simulink model "cartesian_reg"  (Simulink 8.7)
settings: Solver=ode45  StartTime=0.0  StopTime=T  MaxStep=0.01  RelTol=1e-3
values from neighbouring files (symbols this model uses):
  theta_0 = 0    [init.m]
  x_0 = 2    [init.m]
  y_0 = 0    [init.m]
undefined symbols (not defined in the file or in its folder): cart_reg
settings Model: Creator=marilena  LastModifiedBy=giuseppe  ExtModeAutoUpdateStatusClock=off
settings DataIOCC: SignalLoggingSaveFormat=ModelDataLogs
settings OptimizationCC: ExpressionDepthLimit=2147483647
settings DebuggingCC: SaveWithParameterizedLinksMsg=none  SolverPrmCheckMsg=warning  FcnCallInpInsideContextMsg=UseLocalSettings  StateNameClashWarn=warning  StrictBusMsg=Warning
settings HardwareCC: TargetHWDeviceType=32-bit Generic
settings GRTTargetCC: TargetFcnLib=ansi_tfl_tmw.mat  GeneratePreprocessorConditionals=Use local settings  CombineOutputUpdateFcns=off  GRTInterface=on

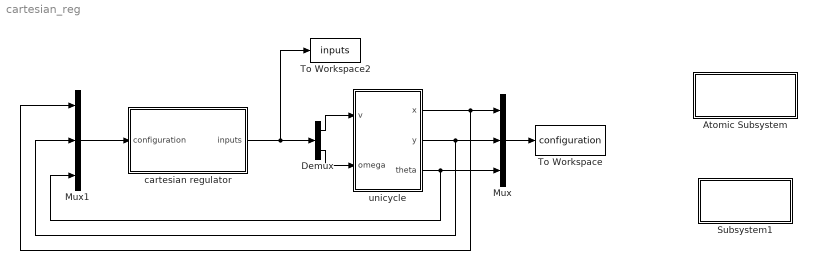
== system cartesian_reg ==
  Atomic Subsystem : Subsystem  TreatAsAtomicUnit=on
      settings: OpenFcn=init
      mask Display: disp('initialization')
  Demux : Demux  Outputs=2
  Mux : Mux  Inputs=3
  Mux1 : Mux  Inputs=3
  Subsystem1 : Subsystem
      settings: OpenFcn=plots
      mask Display: disp('plots')
  To Workspace : ToWorkspace  VariableName=configuration  SaveFormat=Structure With Time  SampleTime=-1
  To Workspace2 : ToWorkspace  VariableName=inputs  SaveFormat=Structure With Time  SampleTime=-1
  cartesian regulator : Subsystem
  unicycle : Subsystem
  wires:
  Mux/1 -> To Workspace/1
  unicycle/3(theta) -> Mux/3, Mux1/3
  unicycle/1(x) -> Mux/1, Mux1/1
  Mux1/1 -> cartesian regulator/1(configuration)
  cartesian regulator/1(inputs) -> Demux/1, To Workspace2/1
  unicycle/2(y) -> Mux/2, Mux1/2
  Demux/1 -> unicycle/1(v)
  Demux/2 -> unicycle/2(omega)

== system cartesian_reg/Atomic Subsystem ==

== system cartesian_reg/Subsystem1 ==

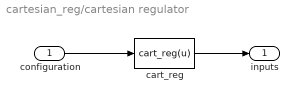
== system cartesian_reg/cartesian regulator ==
  configuration : Inport
  cart_reg : MATLABFcn  Tag={'prova'}  Description=cartesian regulator  MATLABFcn=cart_reg(u)  Output1D=off
  inputs : Outport
  wires:
  configuration/1 -> cart_reg/1
  cart_reg/1 -> inputs/1

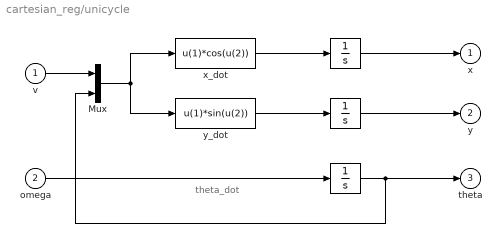
== system cartesian_reg/unicycle ==
  note: theta_dot
  v : Inport
  omega : Inport  Port=2
  " " : Integrator  InitialCondition=theta_0
  "   " : Integrator  InitialCondition=x_0
  "    " : Integrator  InitialCondition=y_0
  Mux : Mux  Inputs=2
  x_dot : Fcn  Expr=u(1)*cos(u(2))
  y_dot : Fcn  Expr=u(1)*sin(u(2))
  x : Outport
  y : Outport  Port=2
  theta : Outport  Port=3
  wires:
  v/1 -> Mux/1
  omega/1 -> " "/1
  x_dot/1 -> "   "/1
  y_dot/1 -> "    "/1
  " "/1 -> Mux/2, theta/1
  Mux/1 -> x_dot/1, y_dot/1
  "   "/1 -> x/1
  "    "/1 -> y/1
